simulink model "sampleModel80"  (R2021b)
settings: Solver=VariableStepAuto  StartTime=0.0  StopTime=10.0  RelTol=1e-3
undefined symbols (not defined in the file or in its folder): DiscIntNeverNeededParam
libraries: simulink x8, slpidlib x1
settings Model: Creator=user  LastModifiedBy=user

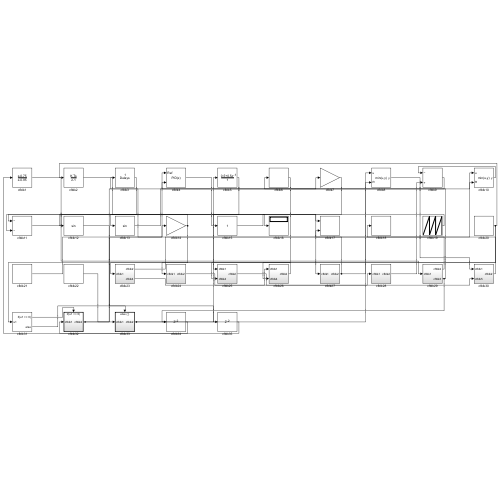
[thumbnail: Simulink's stored preview of the top-level diagram]
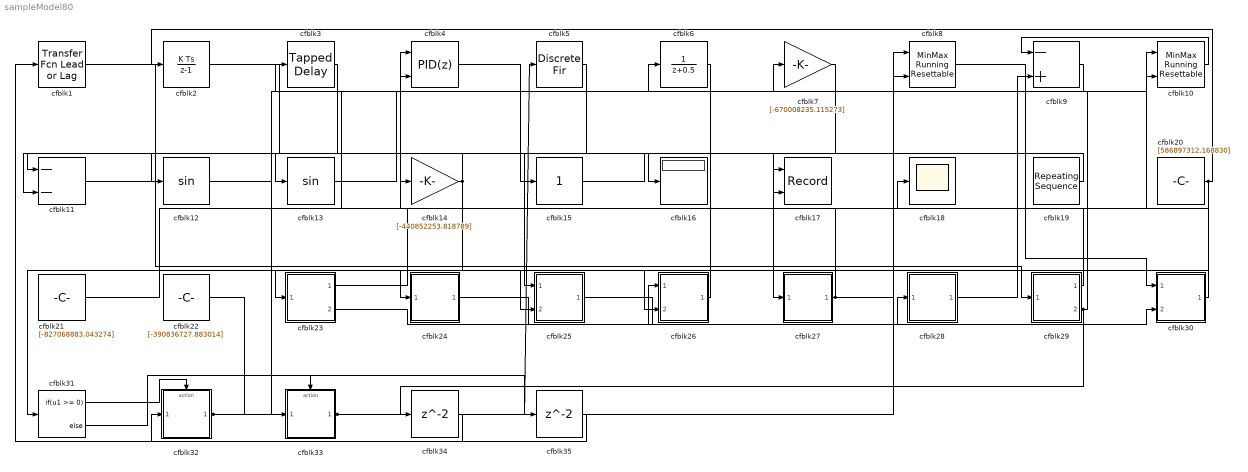
== system sampleModel80 ==
  cfblk1 : simulink/Discrete/Transfer Fcn Lead or Lag  PoleZ=0.95  ZeroZ=0.75  ICPrevOutput=0.0  ICPrevInput=0.0  DoSatur=off
      settings: SourceProductBaseCode=SL
  cfblk10 : simulink/Math Operations/MinMax Running Resettable  Function=min  vinit=0.0
  cfblk11 : Sum  Inputs=--
  cfblk12 : Trigonometry
  cfblk13 : Trigonometry
  cfblk14 : Gain  Gain=[-440852253.818789]
  cfblk15 : simulink/Math Operations/Slider Gain  gain=1  low=0  high=2
  cfblk16 : Display
  cfblk17 : Record  FileSettingsInternal="{\"entries\":[{\"content\":{\"excelSettings\":{\"content\":{},\"type\":\"Streamout.ExcelSettings\"}},\"type\":\"Streamout.FileSettingStorage\",\"uuid\":\"5e234d35-0a2e-4e5e-aa60-8b8856ce2c31\"}],\"packageUris\":[\"http://schema.mathworks.com/mf0/streamout_blocks/R2020a\"],\"version\":\"1.0\"}"  Layout=[1 1]  SignalsInternal="{\"entries\":[{\"content\":{\"signals\":[{\"content\":{\"blockPath\":[\"sampleModel80/cfblk17\"],\"channel\":[],\"dimensions\":[1],\"domain\":\"sampleModel80/cfblk17\",\"lineColor\":\"#a2142f\",\"plots\":[1],\"port\":1,\"sid\":[\"\"],\"signalID\":2974,\"signalName\":\"cfblk15\"},\"type\":\"RecordBlkView.Signal\",\"uuid\":\"e7802b0b-cef9-4407-aa7c-304ea8c3baf8\"},{\"content\":{\"blockPath\":[\"sampleModel80/cfblk17\"],\"channel\":[],\"dimensions\":[1],\"domain\":\"sampleModel80/cfblk17\",\"lineColor\":\"#139fff\",\"plots\":[1],\"port\":2,\"sid\":[\"\"],\"signalID\":2978,\"signalName\":\"cfblk27\"},\"type\":\"RecordBlkView.Signal\",\"uuid\":\"029c59db-96e4-4de6-a270-04919afd9acd\"}]},\"type\":\"RecordBlkView.InputSignals\",\"uuid\":\"2d78a7a5-48fa-474d-8fa8-518c4ce42e45\"}],\"packageUris\":[\"http://schema.mathworks.com/mf0/streamout_blocks/R2020a\"],\"version\":\"1.0\"}"  VisualizationBindings="{\"xyplotplugin\":{\"info\":[{\"series\":[{\"bindingParametersList\":[{\"parameter\":\"X-Axis\",\"signalID\":2974,\"signalName\":\"cfblk15\"},{\"parameter\":\"Y-Axis\",\"signalID\":2978,\"signalName\":\"cfblk27\"}],\"seriesID\":18655}],\"subplotID\":1}]}}"  CompatibilityTag=XY
  cfblk18 : Scope
  cfblk19 : simulink/Sources/Repeating Sequence  rep_seq_t=[0 2]  rep_seq_y=[-923733.214898, 398594216.577377]
  cfblk2 : DiscreteIntegrator  ICPrevOutput=DiscIntNeverNeededParam  ICPrevScaledInput=DiscIntNeverNeededParam
  cfblk20 : Constant  Value=[586897312.168830]  SampleTime=1
  cfblk21 : Constant  Value=[-827068883.043274]  SampleTime=1
  cfblk22 : Constant  Value=[-390836727.883014]  SampleTime=1
  cfblk23 : Subsystem
  cfblk24 : Subsystem
  cfblk25 : Subsystem
  cfblk26 : Subsystem
  cfblk27 : Subsystem
  cfblk28 : Subsystem
  cfblk29 : Subsystem
  cfblk3 : simulink/Discrete/Tapped Delay  vinit=0.0  samptime=-1  NumDelays=1  DelayOrder=Oldest  includeCurrent=off
  cfblk30 : Subsystem
  cfblk31 : If  IfExpression=u1 >= 0  SampleTime=1
  cfblk32 : Subsystem  TreatAsAtomicUnit=on
  cfblk33 : Subsystem  TreatAsAtomicUnit=on
  cfblk34 : Delay  SampleTime=1
  cfblk35 : Delay  SampleTime=1
  cfblk4 : slpidlib/PID Controller (2DOF)  Controller=PID  Form=Parallel  TimeDomain=Discrete-time  UseExternalTs=off  SampleTime=1  IntegratorMethod=Forward Euler  FilterMethod=Forward Euler  ControllerParametersSource=internal  P=1  I=1  D=0  UseFilter=on  N=100  b=1  c=1  TunerSelectOption=Transfer Function Based (PID Tuner App)  InitialConditionSource=internal  InitialConditionForIntegrator=0  InitialConditionForFilter=0  DifferentiatorICPrevScaledInput=0  ExternalReset=none  TrackingMode=off  Kt=1  LimitOutput=off  SatLimitsSource=internal  UpperSaturationLimit=inf  LowerSaturationLimit=-inf  LinearizeAsGain=off  AntiWindupMode=none  Kb=1  POutMin=[]  POutMax=[]  IOutMin=[]  IOutMax=[]  DOutMin=[]  DOutMax=[]  NOutMin=[]  NOutMax=[]  bOutMin=[]  bOutMax=[]  cOutMin=[]  cOutMax=[]  SumOutMin=[]  SumOutMax=[]  SaturationOutMin=[]  SaturationOutMax=[]  PParamMin=[]  PParamMax=[]  IParamMin=[]  IParamMax=[]  DParamMin=[]  DParamMax=[]  NParamMin=[]  NParamMax=[]  bParamMin=[]  bParamMax=[]  cParamMin=[]  cParamMax=[]  KbParamMin=[]  KbParamMax=[]  KtParamMin=[]  KtParamMax=[]  KbOutMin=[]  KbOutMax=[]  KtOutMin=[]  KtOutMax=[]  IntegratorOutMin=[]  IntegratorOutMax=[]  FilterOutMin=[]  FilterOutMax=[]  SumI1OutMin=[]  SumI1OutMax=[]  SumI2OutMin=[]  SumI2OutMax=[]  SumI3OutMin=[]  SumI3OutMax=[]  SumI4OutMin=[]  SumI4OutMax=[]  SumDOutMin=[]  SumDOutMax=[]  Sum1OutMin=[]  Sum1OutMax=[]  Sum2OutMin=[]  Sum2OutMax=[]  Sum3OutMin=[]  Sum3OutMax=[]  DifferentiatorOutMin=[]  DifferentiatorOutMax=[]  FilterDiffOutCoefMin=[]  FilterDiffOutCoefMax=[]  ReciprocalOutMin=[]  ReciprocalOutMax=[]  SumDenOutMin=[]  SumDenOutMax=[]  SumNumOutMin=[]  SumNumOutMax=[]  DivideOutMin=[]  DivideOutMax=[]  UdiffTsProdOutMin=[]  UdiffTsProdOutMax=[]  NTsProdOutMin=[]  NTsProdOutMax=[]  UintegralTsProdOutMin=[]  UintegralTsProdOutMax=[]  UngainTsProdOutMin=[]  UngainTsProdOutMax=[]  IntegratorContinuousStateAttributes=''  IntegratorStateMustResolveToSignalObject=off  IntegratorRTWStateStorageClass=Auto  FilterContinuousStateAttributes=''  FilterStateMustResolveToSignalObject=off  FilterRTWStateStorageClass=Auto  ParallelPVariant=InternalParameters  IdealPVariant=Disabled  IVariant=InternalParameters  DVariant=InternalParameters  bVariant=InternalParameters  cVariant=InternalParameters  IntegratorVariant=Discrete  SatVariant=Disabled  AWVariant=Passthrough  PCopyVariant=Disabled  TRVariant=Disabled  FdbkBlocksVariant=Forward  IdealPFdbkVariant=Disabled  SatFdbkVariant=Disabled  DerivativeFilterVariant=ForwardEulerFilter  NVariant=InternalParameters  NCopyVariant=Disabled  FilterICVariant=InternalICsFilter  IntegratorICVariant=InternalICs  ExternalResetVariant=Disabled  TRSumVariant=Passthrough  SumFdbkVariant=Disabled  SumVariant=Sum_PID  TsampFilterVariant=InternalTs  TsampNgainVariant=Passthrough  TsampIntegralVariant=Passthrough  ExternalSaturationOutDataTypeStr=Inherit: Same as second input
      settings: SourceProductBaseCode=SL
  cfblk5 : DiscreteFir  SampleTime=1
  cfblk6 : DiscreteTransferFcn  SampleTime=1
  cfblk7 : Gain  Gain=[-670008235.115273]
  cfblk8 : simulink/Math Operations/MinMax Running Resettable  Function=min  vinit=0.0
  cfblk9 : Sum  Inputs=-+
  wires:
  cfblk22/1 -> cfblk33/1(cfblk1)
  cfblk26/1(cfblk2) -> cfblk31/1
  cfblk1/1 -> cfblk29/1(cfblk1)
  cfblk8/1 -> cfblk30/1(cfblk1)
  cfblk33/1(cfblk2) -> cfblk5/1, cfblk8/2
  cfblk3/1 -> cfblk13/1
  cfblk2/1 -> cfblk27/1(cfblk1)
  cfblk25/1(cfblk2) -> cfblk28/1(cfblk1)
  cfblk23/1(cfblk2) -> cfblk10/1
  cfblk10/1 -> cfblk9/1
  cfblk5/1 -> cfblk25/1(cfblk1)
  cfblk23/2(cfblk4) -> cfblk26/1(cfblk1)
  cfblk21/1 -> cfblk4/1
  cfblk19/1 -> cfblk11/1
  cfblk20/1 -> cfblk2/1, cfblk25/2(cfblk4), cfblk26/2(cfblk4)
  cfblk7/1 -> cfblk11/2
  cfblk9/1 -> cfblk4/2
  cfblk24/1(cfblk2) -> cfblk30/2(cfblk5)
  cfblk30/1(cfblk2) -> cfblk3/1
  cfblk32/1(cfblk2) -> cfblk14/1, cfblk10/2
  cfblk13/1 -> cfblk7/1
  cfblk29/1(cfblk2) -> cfblk18/1
  cfblk4/1 -> cfblk15/1
  cfblk6/1 -> cfblk23/1(cfblk1)
  cfblk29/2(cfblk3) -> cfblk6/1, cfblk34/1
  cfblk28/1(cfblk2) -> cfblk9/2
  cfblk27/1(cfblk2) -> cfblk8/1, cfblk17/2
  cfblk11/1 -> cfblk16/1
  cfblk14/1 -> cfblk12/1, cfblk24/1(cfblk1)
  cfblk15/1 -> cfblk17/1
  cfblk31/1 -> cfblk32/Action
  cfblk31/2 -> cfblk33/Action
  cfblk34/1 -> cfblk1/1
  cfblk12/1 -> cfblk35/1
  cfblk35/1 -> cfblk32/1(cfblk1)

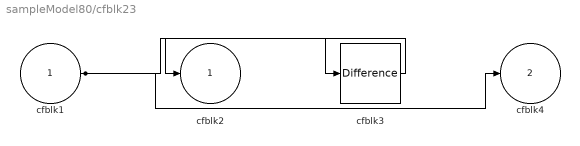
== system sampleModel80/cfblk23 ==
  cfblk1 : Inport
  cfblk3 : simulink/Discrete/Difference  ICPrevInput=0.0  OutMin=[]  OutMax=[]  OutDataTypeStr=Inherit: Inherit via back propagation  OutDataType=fixdt(1, 16)  OutScaling=2^-10  DoSatur=off
  cfblk2 : Outport
  cfblk4 : Outport  Port=2
  wires:
  cfblk3/1 -> cfblk2/1
  cfblk1/1 -> cfblk4/1, cfblk3/1

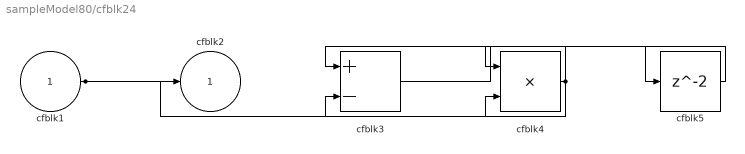
== system sampleModel80/cfblk24 ==
  cfblk1 : Inport
  cfblk3 : Sum  Inputs=+-
  cfblk4 : Product  Inputs=**
  cfblk5 : Delay  SampleTime=1
  cfblk2 : Outport
  wires:
  cfblk4/1 -> cfblk3/1, cfblk3/2
  cfblk1/1 -> cfblk2/1, cfblk4/2
  cfblk3/1 -> cfblk5/1
  cfblk5/1 -> cfblk4/1

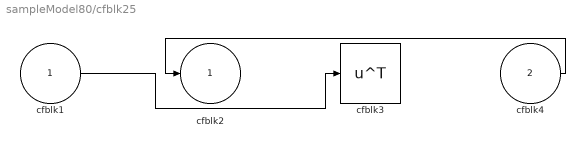
== system sampleModel80/cfblk25 ==
  cfblk1 : Inport
  cfblk4 : Inport  Port=2
  cfblk3 : Math  Operator=transpose  SaturateOnIntegerOverflow=on
  cfblk2 : Outport
  wires:
  cfblk4/1 -> cfblk2/1
  cfblk1/1 -> cfblk3/1

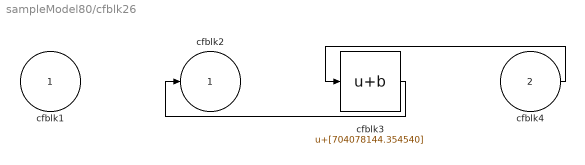
== system sampleModel80/cfblk26 ==
  cfblk1 : Inport
  cfblk4 : Inport  Port=2
  cfblk3 : Bias  Bias=[704078144.354540]
  cfblk2 : Outport
  wires:
  cfblk4/1 -> cfblk3/1
  cfblk3/1 -> cfblk2/1

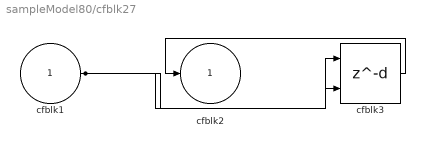
== system sampleModel80/cfblk27 ==
  cfblk1 : Inport
  cfblk3 : Delay  DelayLengthSource=Input port  SampleTime=1
      settings: InputPortMap=u0,p1
  cfblk2 : Outport
  wires:
  cfblk3/1 -> cfblk2/1
  cfblk1/1 -> cfblk3/1, cfblk3/2

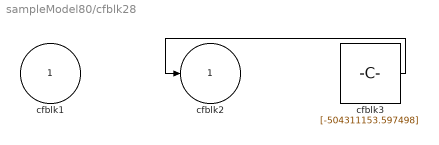
== system sampleModel80/cfblk28 ==
  cfblk1 : Inport
  cfblk3 : Constant  Value=[-504311153.597498]  SampleTime=1
  cfblk2 : Outport
  wires:
  cfblk3/1 -> cfblk2/1

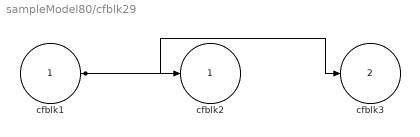
== system sampleModel80/cfblk29 ==
  cfblk1 : Inport
  cfblk2 : Outport
  cfblk3 : Outport  Port=2
  wires:
  cfblk1/1 -> cfblk2/1, cfblk3/1

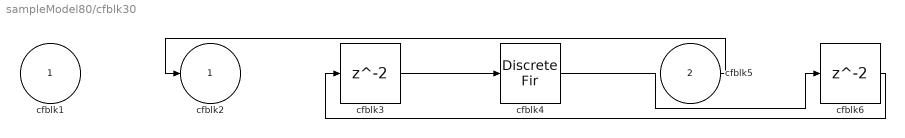
== system sampleModel80/cfblk30 ==
  cfblk1 : Inport
  cfblk5 : Inport  Port=2
  cfblk3 : Delay  SampleTime=1
  cfblk4 : DiscreteFir  SampleTime=1
  cfblk6 : Delay  SampleTime=1
  cfblk2 : Outport
  wires:
  cfblk5/1 -> cfblk2/1
  cfblk3/1 -> cfblk4/1
  cfblk4/1 -> cfblk6/1
  cfblk6/1 -> cfblk3/1

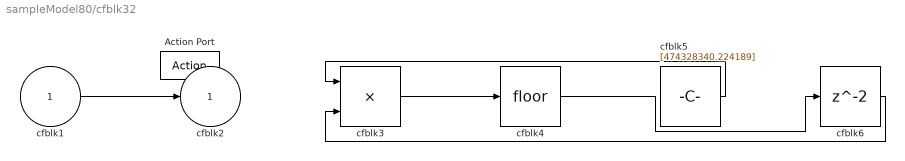
== system sampleModel80/cfblk32 ==
  cfblk1 : Inport
  Action Port : ActionPort  ActionPortLabel=if(u1 >= 0)
  cfblk3 : Product  Inputs=**
  cfblk4 : Rounding
  cfblk5 : Constant  Value=[474328340.224189]  SampleTime=1
  cfblk6 : Delay
  cfblk2 : Outport
  wires:
  cfblk3/1 -> cfblk4/1
  cfblk5/1 -> cfblk3/1
  cfblk1/1 -> cfblk2/1
  cfblk4/1 -> cfblk6/1
  cfblk6/1 -> cfblk3/2

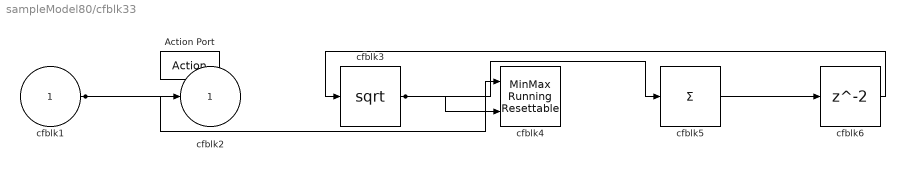
== system sampleModel80/cfblk33 ==
  cfblk1 : Inport
  Action Port : ActionPort  ActionPortLabel=else
  cfblk3 : Sqrt  SaturateOnIntegerOverflow=on
  cfblk4 : simulink/Math Operations/MinMax Running Resettable  Function=min  vinit=0.0
  cfblk5 : Sum  Inputs=+
  cfblk6 : Delay
  cfblk2 : Outport
  wires:
  cfblk3/1 -> cfblk5/1, cfblk4/2
  cfblk1/1 -> cfblk2/1, cfblk4/1
  cfblk5/1 -> cfblk6/1
  cfblk6/1 -> cfblk3/1
